simulink model "AIE_HLS_8_32"  (R2019b)
settings: Solver=VariableStepAuto  StartTime=0.0  StopTime=100  RelTol=1e-3
undefined symbols (not defined in the file): xc7vx485tffg1157
libraries: ModelComposer x8, simulink x1
settings Model: Creator=viswanad  LastModifiedBy=abehbood
settings DataIOCC: ReturnWorkspaceOutputs=off
settings SFSimCC: CustomCodeUndefinedFunction=UseInterfaceOnly

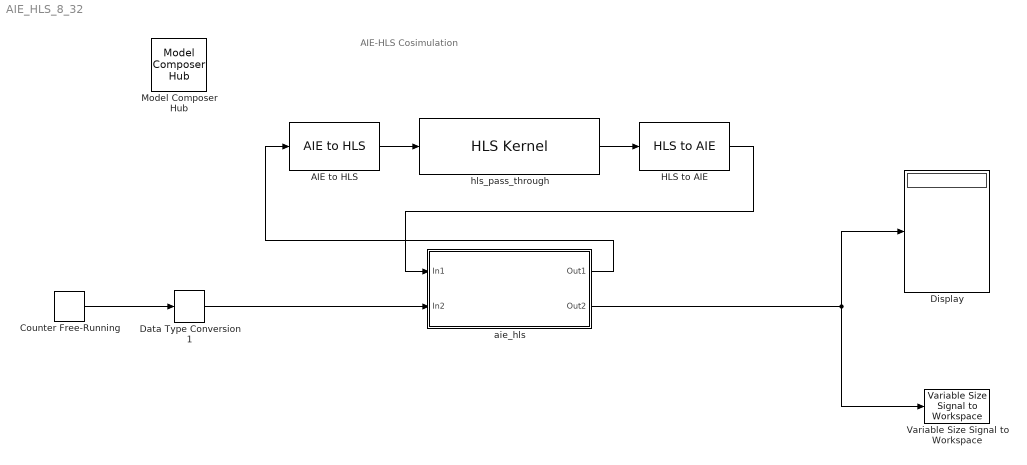
== system AIE_HLS_8_32 ==
  note: AIE-HLS Cosimulation
  AIE to HLS : ModelComposer/AIE to HLS  OutputType=ap_axis<32,0,0,0>  OutputSize=1
  Counter Free-Running : simulink/Sources/Counter Free-Running  NumBits=8  tsamp=1
  Data Type Conversion1 : ModelComposer/Data Type Conversion  OutDataType=int8  TypeExp=''  Signedness=Signed  WordLength=64  FractionalLength=0  RoundingMode=Truncation to minus infinity  OverflowMode=Wrap around
  Display : Display
  HLS to AIE : ModelComposer/HLS to AIE  OutputType=int8  OutputSize=4
  Model Composer Hub : ModelComposer/Model Composer Hub  CodeGeneration=off  SubsystemName=aie_hls  TargetDirectory=./aie_hls_8_32  ExportType=AI Engines  IpVendor=xilinx.com  IpLibrary=hls  IpVersion=1.0  IpHWLanguage=Verilog  AieCompilerOptions={}  CreateTestbench=on  TestbenchStackSize=10  RunAieSim=on  AieSimTimeout=5000  LaunchVitisAnalyzer=off  RunX86Sim=off  X86SimTimeout=10  ProjDevice=xc7vx485tffg1157-1  ProjDevicePart=xc7vx485tffg1157-1  SamplePeriod=-1  ClockFrequency=200  DataPathParallelism=1
  Variable Size Signal to Workspace : ModelComposer/Variable Size Signal to Workspace  VariableNameMask=simout
  aie_hls : Subsystem
  hls_pass_through : ModelComposer/HLS Kernel  PortAttributesTable={ 'Input', 'in_sample', 'adf::dir::in< hls::stream< hls::axis< ap_int< 32 >, 0, 0, 0 >, 0 > & >', '', ''; 'Output', 'out_sample', 'adf::dir::out< hls::stream< hls::axis< ap_int< 32 >, 0, 0, 0 >, 0 > & >', '', '1' }  PortAttributesEnablement={'off', 'off', 'off', 'off', 'off';'off', 'off', 'off', 'off', 'on'}  FormalArgDecls={'adf::dir::in< hls::stream< hls::axis< ap_int< 32 >, 0, 0, 0 >, 0 > & > in_sample', 'adf::dir::out< hls::stream< hls::axis< ap_int< 32 >, 0, 0, 0 >, 0 > & > out_sample'}  PortSynchronicities={'auto'; 'auto'}  PortSignalSizes={0.000000000000000000e+00; 1.000000000000000000e+00}  SimLibPath=''  FunctionTabVisible=on  FunctionDescription=void hls_pass_through(adf::dir::in< hls::stream< hls::axis< ap_int< 32 >, 0, 0, 0 >, 0 > & > in_sample, adf::dir::out< hls::stream< hls::axis< ap_int< 32 >, 0, 0, 0 >, 0 > & > out_sample)  KernelHeaderFile=src/8_32_bit/hls_kernel.h  KernelFunction=hls_pass_through  KernelFunctionSelect=<empty>  KernelSourceFile=src/8_32_bit/hls_pass_through.cpp  KernelSearchPaths={}  PreProcOptions={}
  wires:
  Counter Free-Running/1 -> Data Type Conversion1/1
  AIE to HLS/1 -> hls_pass_through/1
  hls_pass_through/1 -> HLS to AIE/1
  aie_hls/2(Out2) -> Variable Size Signal to Workspace/1, Display/1
  HLS to AIE/1 -> aie_hls/1(In1)
  Data Type Conversion1/1 -> aie_hls/2(In2)
  aie_hls/1(Out1) -> AIE to HLS/1

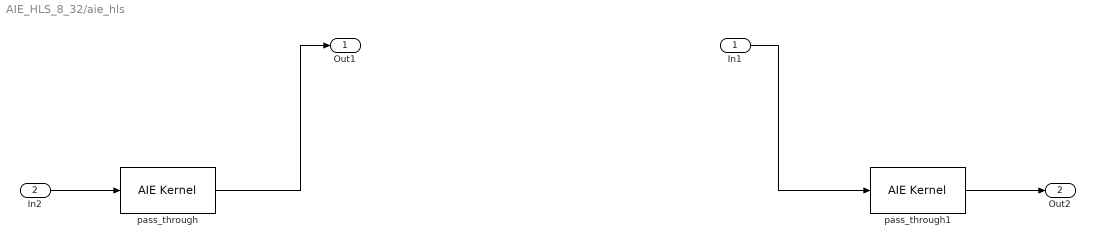
== system AIE_HLS_8_32/aie_hls ==
  In1 : Inport
  In2 : Inport  Port=2
  pass_through : ModelComposer/AIE Kernel  PortAttributesTable={ 'Input', 'in', 'input_stream_int8 *', '', '', '', ''; 'Output', 'out', 'output_stream_int8 *', '', '', '', '4' }  PortAttributesEnablement={'off', 'off', 'off', 'off', 'off', 'off', 'off';'off', 'off', 'off', 'off', 'off', 'off', 'on'}  FormalArgDecls={'input_stream_int8 * in', 'output_stream_int8 * out'}  PortWindowSizes={0.000000000000000000e+00; 0.000000000000000000e+00}  PortWindowMargins={0.000000000000000000e+00; 0.000000000000000000e+00}  PortSynchronicities={'auto'; 'auto'}  PortSignalSizes={0.000000000000000000e+00; 4.000000000000000000e+00}  SimLibPath=''  FunctionTabVisible=on  FunctionDescription=void pass_through(input_stream_int8 * in, output_stream_int8 * out)  KernelHeaderFile=src/8_32_bit/aie_pass_through.h  KernelFunction=pass_through  KernelFunctionSelect=<empty>  KernelSourceFile=src/8_32_bit/aie_pass_through.cc  KernelSearchPaths={}  PreProcOptions={}  CoreRuntimeRatio=0.9  KernelLocSpec=off  ColRowLocation=[0 0]
  pass_through1 : ModelComposer/AIE Kernel  PortAttributesTable={ 'Input', 'in', 'input_stream_int8 *', '', '', '', ''; 'Output', 'out', 'output_stream_int8 *', '', '', '', '1' }  PortAttributesEnablement={'off', 'off', 'off', 'off', 'off', 'off', 'off';'off', 'off', 'off', 'off', 'off', 'off', 'on'}  FormalArgDecls={'input_stream_int8 * in', 'output_stream_int8 * out'}  PortWindowSizes={0.000000000000000000e+00; 0.000000000000000000e+00}  PortWindowMargins={0.000000000000000000e+00; 0.000000000000000000e+00}  PortSynchronicities={'auto'; 'auto'}  PortSignalSizes={0.000000000000000000e+00; 1.000000000000000000e+00}  SimLibPath=''  FunctionTabVisible=on  FunctionDescription=void pass_through(input_stream_int8 * in, output_stream_int8 * out)  KernelHeaderFile=src/8_32_bit/aie_pass_through.h  KernelFunction=pass_through  KernelFunctionSelect=<empty>  KernelSourceFile=src/8_32_bit/aie_pass_through.cc  KernelSearchPaths={}  PreProcOptions={}  CoreRuntimeRatio=0.9  KernelLocSpec=off  ColRowLocation=[0 0]
  Out1 : Outport
  Out2 : Outport  Port=2
  wires:
  pass_through/1 -> Out1/1
  In1/1 -> pass_through1/1
  pass_through1/1 -> Out2/1
  In2/1 -> pass_through/1
